simulink model "WTxPSMG3"  (R2023b)
settings: Solver=FixedStepAuto  StartTime=0.0  StopTime=0.2  FixedStep=0.000001  RelTol=1e-3
undefined symbols (not defined in the file): c1, c2, c3, c5, c6, J, Ke, lambda_opt, Ld, Lq, omega_r, p, R, ro, Rs
libraries: slpidlib x1, simulink x1
settings Model: Creator=tudorn  LastModifiedBy=tudorn

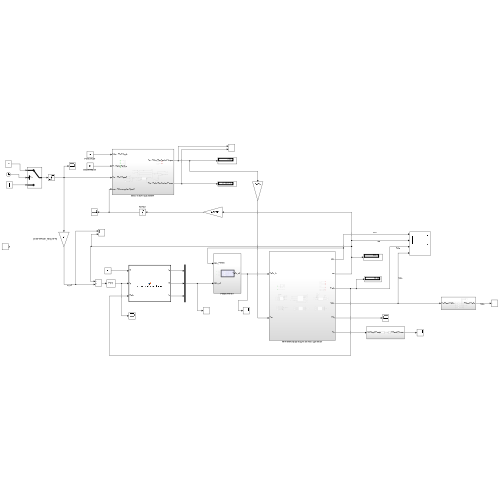
[thumbnail: Simulink's stored preview of the top-level diagram]
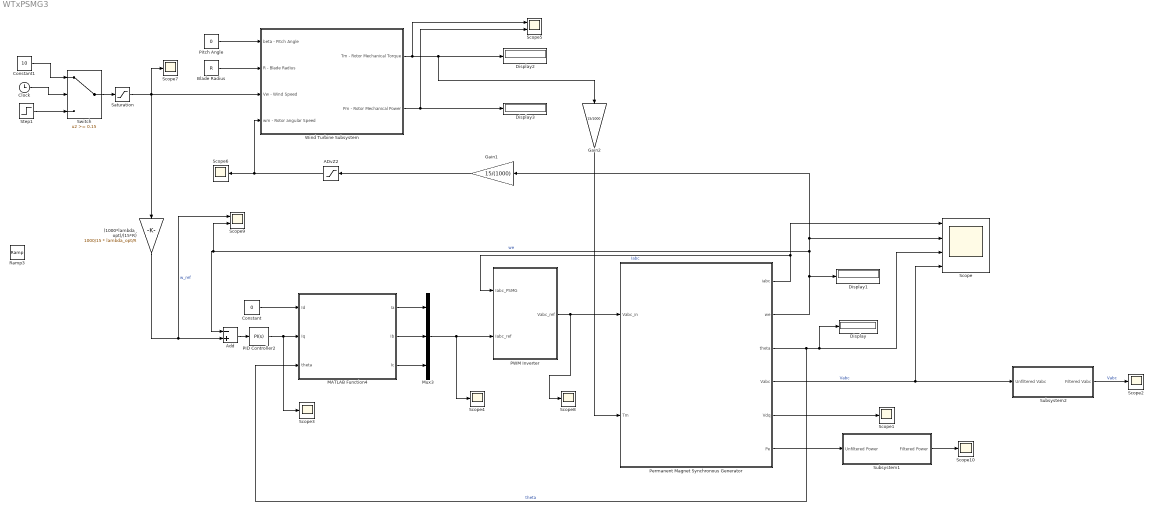
== system WTxPSMG3 ==
  (1000*lambda_opt)/(15*R) : Gain  Gain=1000/15 * lambda_opt/R
  ADvZ2 : Saturate  UpperLimit=omega_r  LowerLimit=1e-6
  Add : Sum  Inputs=-+
  Blade Radius : Constant  Value=R
  Clock : Clock
  Constant : Constant  Value=0
  Constant1 : Constant  Value=10
  Display{,1..3} (4 alike) : Display
  Gain1 : Gain  Gain=15/(1000)
  Gain2 : Gain  Gain=15/1000
  MATLAB Function4 : MATLAB Function  TreatAsAtomicUnit=on
  Mux3 : Mux  Inputs=3
  PID Controller2 : slpidlib/PID Controller  Controller=PI  Form=Parallel  TimeDomain=Continuous-time  UseExternalTs=off  SampleTime=-1  IntegratorMethod=Forward Euler  FilterMethod=Forward Euler  ControllerParametersSource=internal  P=40  I=3  UseKiTs=off  D=0  N=100  UseFilter=on  TunerSelectOption=Transfer Function Based (PID Tuner App)  InitialConditionSource=internal  InitialConditionForIntegrator=0  InitialConditionForFilter=0  DifferentiatorICPrevScaledInput=0  ExternalReset=none  TrackingMode=off  Kt=1  LimitOutput=off  SatLimitsSource=internal  UpperSaturationLimit=inf  LowerSaturationLimit=-inf  LinearizeAsGain=on  AntiWindupMode=none  Kb=1  LimitIntegrator=off  UpperIntegratorSaturationLimit=inf  LowerIntegratorSaturationLimit=-inf  POutMin=[]  POutMax=[]  IOutMin=[]  IOutMax=[]  DOutMin=[]  DOutMax=[]  NOutMin=[]  NOutMax=[]  SumOutMin=[]  SumOutMax=[]  SaturationOutMin=[]  SaturationOutMax=[]  PParamMin=[]  PParamMax=[]  IParamMin=[]  IParamMax=[]  DParamMin=[]  DParamMax=[]  NParamMin=[]  NParamMax=[]  KbParamMin=[]  KbParamMax=[]  KtParamMin=[]  KtParamMax=[]  KbOutMin=[]  KbOutMax=[]  KtOutMin=[]  KtOutMax=[]  IntegratorOutMin=[]  IntegratorOutMax=[]  FilterOutMin=[]  FilterOutMax=[]  SumI1OutMin=[]  SumI1OutMax=[]  SumI2OutMin=[]  SumI2OutMax=[]  SumI3OutMin=[]  SumI3OutMax=[]  SumI4OutMin=[]  SumI4OutMax=[]  SumDOutMin=[]  SumDOutMax=[]  DifferentiatorOutMin=[]  DifferentiatorOutMax=[]  FilterDiffOutCoefMin=[]  FilterDiffOutCoefMax=[]  ReciprocalOutMin=[]  ReciprocalOutMax=[]  SumDenOutMin=[]  SumDenOutMax=[]  SumNumOutMin=[]  SumNumOutMax=[]  DivideOutMin=[]  DivideOutMax=[]  UdiffTsProdOutMin=[]  UdiffTsProdOutMax=[]  NTsProdOutMin=[]  NTsProdOutMax=[]  UintegralTsProdOutMin=[]  UintegralTsProdOutMax=[]  UngainTsProdOutMin=[]  UngainTsProdOutMax=[]  ClampingZeroOutDataTypeStr=Inherit: Inherit via back propagation  ClampingZeroOutMin=[]  ClampingZeroOutMax=[]  FilterDenConstantOutDataTypeStr=Inherit: Inherit via back propagation  FilterDenConstantOutMin=[]  FilterDenConstantOutMax=[]  PCopyOutDataTypeStr=Inherit: Inherit via back propagation  PCopyOutMin=[]  PCopyOutMax=[]  NCopyOutDataTypeStr=Inherit: Inherit via back propagation  NCopyOutMin=[]  NCopyOutMax=[]  IntegratorContinuousStateAttributes=''  IntegratorStateMustResolveToSignalObject=off  IntegratorRTWStateStorageClass=Auto  FilterContinuousStateAttributes=''  FilterStateMustResolveToSignalObject=off  FilterRTWStateStorageClass=Auto  ParallelPVariant=InternalParameters  IdealPVariant=Disabled  IVariant=InternalParameters  DVariant=Disabled  IntegratorVariant=Continuous  SatVariant=Disabled  AWVariant=Passthrough  PCopyVariant=Disabled  TRVariant=Disabled  FdbkBlocksVariant=Forward  IdealPFdbkVariant=Disabled  SatFdbkVariant=Disabled  DerivativeFilterVariant=Disabled  NVariant=Disabled  NCopyVariant=Disabled_SignalSpec  FilterICVariant=Disabled  IntegratorICVariant=InternalICs  ExternalResetVariant=Disabled  TRSumVariant=Passthrough  SumFdbkVariant=Disabled  SumVariant=Sum_PI  TsampFilterVariant=InternalTs  TsampNgainVariant=Passthrough  TsampIntegralVariant=Disabled_SignalSpec  ExternalSaturationOutDataTypeStr=Inherit: Same as second input
  PWM Inverter : Subsystem
  Permanent Magnet Synchronous Generator : Subsystem
  Pitch Angle : Constant  Value=0
  Ramp3 : simulink/Sources/Ramp  slope=100  start=0.02  InitialOutput=7
  Saturation : Saturate  UpperLimit=13  LowerLimit=0
  Scope : Scope  NumInputPorts=4
  Scope{1..4,6..8,10} (8 alike) : Scope
  Scope5 : Scope  NumInputPorts=2
  Scope9 : Scope  NumInputPorts=2
  Step1 : Step  Time=0.075  Before=7  After=12  SampleTime=0
  Subsystem1 : Subsystem
  Subsystem2 : Subsystem
  Switch : Switch  Threshold=0.15  SaturateOnIntegerOverflow=off  InputSameDT=off
  Wind Turbine Subsystem : Subsystem
  wires:
  Gain2/1 -> Permanent Magnet Synchronous Generator/2(Tm)
  PWM Inverter/1(Vabc_ref) -> Scope8/1, Permanent Magnet Synchronous Generator/1(Vabc_in)
  Gain1/1 -> ADvZ2/1
  Blade Radius/1 -> Wind Turbine Subsystem/2(R - Blade Radius)
  MATLAB Function4/1(Ia) -> Mux3/1
  MATLAB Function4/2(Ib) -> Mux3/2
  Constant/1 -> MATLAB Function4/1(Id)
  Pitch Angle/1 -> Wind Turbine Subsystem/1(beta - Pitch Angle)
  Mux3/1 -> Scope4/1, PWM Inverter/2(Iabc_ref)
  Saturation/1 -> Wind Turbine Subsystem/3(Vw - Wind Speed), Scope7/1, (1000*lambda_opt)/(15*R)/1
  Wind Turbine Subsystem/2(Pm - Rotor Mechanical Power) -> Display3/1, Scope5/2
  Wind Turbine Subsystem/1(Tm - Rotor Mechanical Torque) -> Gain2/1, Display2/1, Scope5/1
  Permanent Magnet Synchronous Generator/1(iabc) -> Scope/1, PWM Inverter/1(Iabc_PSMG)  "Iabc"
  MATLAB Function4/3(Ic) -> Mux3/3
  Permanent Magnet Synchronous Generator/3(theta) -> MATLAB Function4/3(theta), Display/1, Scope/3  "theta"
  Permanent Magnet Synchronous Generator/2(we) -> Scope9/2, Add/1, Scope/2, Gain1/1, Display1/1  "we"
  (1000*lambda_opt)/(15*R)/1 -> Add/2, Scope9/1  "w_ref"
  Permanent Magnet Synchronous Generator/5(Vdq) -> Scope1/1
  ADvZ2/1 -> Scope6/1, Wind Turbine Subsystem/4(wm - Rotor angular Speed)
  Permanent Magnet Synchronous Generator/4(Vabc) -> Subsystem2/1(Unfiltered Vabc), Scope/4  "Vabc"
  Add/1 -> PID Controller2/1
  PID Controller2/1 -> Scope3/1, MATLAB Function4/2(Iq)
  Permanent Magnet Synchronous Generator/6(Pe) -> Subsystem1/1(Unfiltered Power)
  Subsystem2/1(Filtered Vabc) -> Scope2/1  "Vabc"
  Subsystem1/1(Filtered Power) -> Scope10/1
  Switch/1 -> Saturation/1
  Constant1/1 -> Switch/1
  Step1/1 -> Switch/3
  Clock/1 -> Switch/2

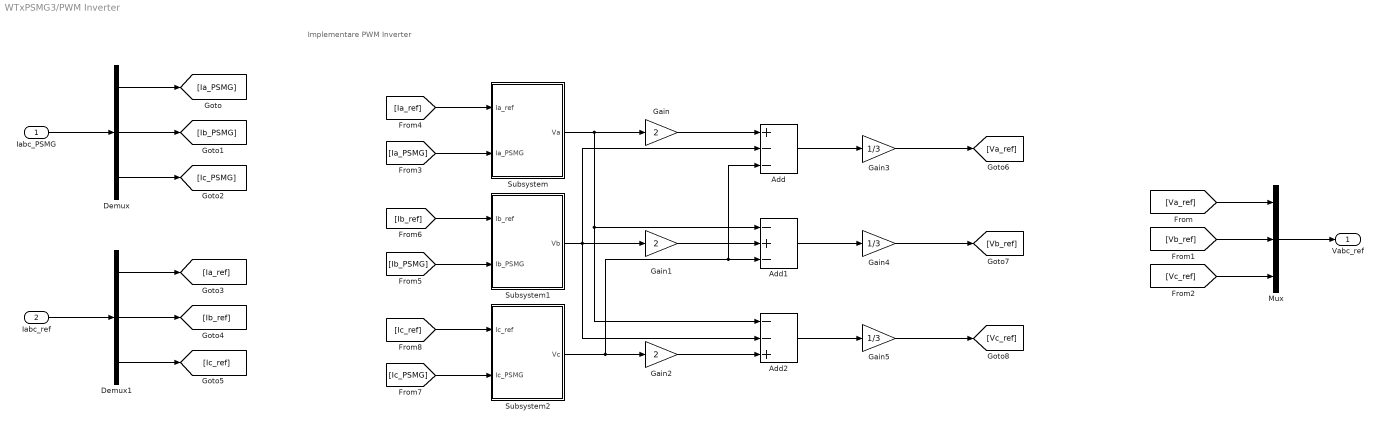
== system WTxPSMG3/PWM Inverter ==
  note: Implementare PWM Inverter
  Iabc_PSMG : Inport
  Iabc_ref : Inport  Port=2
  Add : Sum  Inputs=+--
  Add1 : Sum  Inputs=-+-
  Add2 : Sum  Inputs=--+
  Demux : Demux  Outputs=3
  Demux1 : Demux  Outputs=3
  Gain : Gain  Gain=2
  Gain1 : Gain  Gain=2
  Gain2 : Gain  Gain=2
  Gain3 : Gain  Gain=1/3
  Gain4 : Gain  Gain=1/3
  Gain5 : Gain  Gain=1/3
  Mux : Mux  Inputs=3
  Subsystem : Subsystem
  Subsystem1 : Subsystem
  Subsystem2 : Subsystem
  Vabc_ref : Outport
  wires:
  Iabc_PSMG/1 -> Demux/1
  Mux/1 -> Vabc_ref/1
  Demux/1 -> [Ia_PSMG]
  Demux/2 -> [Ib_PSMG]
  Demux/3 -> [Ic_PSMG]
  Demux1/3 -> [Ic_ref]
  Demux1/2 -> [Ib_ref]
  Demux1/1 -> [Ia_ref]
  Iabc_ref/1 -> Demux1/1
  [Va_ref] -> Mux/1
  [Vb_ref] -> Mux/2
  [Vc_ref] -> Mux/3
  [Ia_ref] -> Subsystem/1(Ia_ref)
  [Ia_PSMG] -> Subsystem/2(Ia_PSMG)
  [Ib_ref] -> Subsystem1/1(Ib_ref)
  [Ib_PSMG] -> Subsystem1/2(Ib_PSMG)
  [Ic_ref] -> Subsystem2/1(Ic_ref)
  [Ic_PSMG] -> Subsystem2/2(Ic_PSMG)
  Subsystem/1(Va) -> Add2/1, Add1/1, Gain/1
  Subsystem2/1(Vc) -> Add/3, Add1/3, Gain2/1
  Subsystem1/1(Vb) -> Add2/2, Gain1/1, Add/2
  Gain/1 -> Add/1
  Gain1/1 -> Add1/2
  Gain2/1 -> Add2/3
  Add/1 -> Gain3/1
  Add1/1 -> Gain4/1
  Add2/1 -> Gain5/1
  Gain5/1 -> [Vc_ref]
  Gain4/1 -> [Vb_ref]
  Gain3/1 -> [Va_ref]

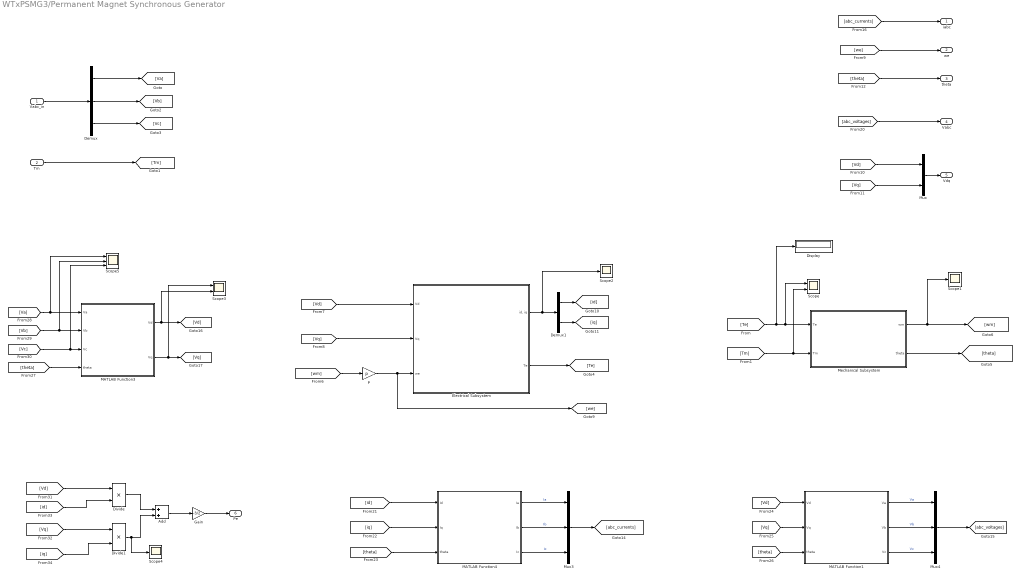
== system WTxPSMG3/Permanent Magnet Synchronous Generator ==
  Vabc_in : Inport
  Tm : Inport  Port=2
  Add : Sum
  Demux : Demux  Outputs=3
  Demux1 : Demux  Outputs=2
  Display : Display
  Divide : Product  Inputs=**
  Divide1 : Product  Inputs=**
  Electrical Subsystem : Subsystem
  Gain : Gain  Gain=-3/2
  MATLAB Function1 : MATLAB Function  TreatAsAtomicUnit=on
  MATLAB Function3 : MATLAB Function  TreatAsAtomicUnit=on
  MATLAB Function4 : MATLAB Function  TreatAsAtomicUnit=on
  Mechanical Subsystem : Subsystem
  Mux : Mux  Inputs=2
  Mux3 : Mux  Inputs=3
  Mux4 : Mux  Inputs=3
  P : Gain  Gain=p
  Scope : Scope  NumInputPorts=2
  Scope1 : Scope
  Scope2 : Scope
  Scope3 : Scope  NumInputPorts=2
  Scope4 : Scope
  Scope5 : Scope  NumInputPorts=3
  iabc : Outport
  we : Outport  Port=2
  theta : Outport  Port=3
  Vabc : Outport  Port=4
  Vdq : Outport  Port=5
  Pe : Outport  Port=6
  wires:
  Vabc_in/1 -> Demux/1
  Tm/1 -> [Tm]
  Demux/1 -> [Va]
  Demux/2 -> [Vb]
  Demux/3 -> [Vc]
  Electrical Subsystem/2(Te) -> [Te]
  [Te] -> Display/1, Scope/1, Mechanical Subsystem/1(Te)
  [Tm] -> Scope/2, Mechanical Subsystem/2(Tm)
  Mechanical Subsystem/1(wm) -> Scope1/1, [wm]
  [wm] -> P/1
  P/1 -> [we], Electrical Subsystem/3(we)
  [Vq] -> Electrical Subsystem/2(Vq)
  [Vd] -> Electrical Subsystem/1(Vd)
  [we] -> we/1
  Mux/1 -> Vdq/1
  [Vd] -> Mux/1
  [Vq] -> Mux/2
  [theta] -> theta/1
  Electrical Subsystem/1("id, iq") -> Scope2/1, Demux1/1
  Demux1/1 -> [id]
  Demux1/2 -> [iq]
  [abc_currents] -> iabc/1
  [abc_voltages] -> Vabc/1
  [iq] -> MATLAB Function4/2(Iq)
  [theta] -> MATLAB Function4/3(theta)
  [id] -> MATLAB Function4/1(Id)
  Mux3/1 -> [abc_currents]
  MATLAB Function4/2(Ib) -> Mux3/2  "Ib"
  MATLAB Function4/1(Ia) -> Mux3/1  "Ia"
  MATLAB Function4/3(Ic) -> Mux3/3  "Ic"
  [Vd] -> MATLAB Function1/1(Vd)
  [Vq] -> MATLAB Function1/2(Vq)
  [theta] -> MATLAB Function1/3(theta)
  Mux4/1 -> [abc_voltages]
  MATLAB Function1/1(Va) -> Mux4/1  "Va"
  MATLAB Function1/2(Vb) -> Mux4/2  "Vb"
  MATLAB Function1/3(Vc) -> Mux4/3  "Vc"
  [Va] -> Scope5/1, MATLAB Function3/1(Va)
  [Vc] -> Scope5/3, MATLAB Function3/3(Vc)
  [theta] -> MATLAB Function3/4(theta)
  [Vb] -> Scope5/2, MATLAB Function3/2(Vb)
  MATLAB Function3/2(Vq) -> Scope3/1, [Vq]
  MATLAB Function3/1(Vd) -> Scope3/2, [Vd]
  [Vq] -> Divide1/1
  [iq] -> Divide1/2
  [id] -> Divide/2
  [Vd] -> Divide/1
  Divide/1 -> Add/1
  Divide1/1 -> Scope4/1, Add/2
  Add/1 -> Gain/1
  Gain/1 -> Pe/1
  Mechanical Subsystem/2(theta) -> [theta]

== system WTxPSMG3/Subsystem1 ==
  Unfiltered Power : Inport
  Saturation : Saturate  UpperLimit=4500  LowerLimit=-45
  Transfer Fcn : TransferFcn  Denominator=[1e-2 1]
  Filtered Power : Outport
  wires:
  Transfer Fcn/1 -> Saturation/1
  Unfiltered Power/1 -> Transfer Fcn/1
  Saturation/1 -> Filtered Power/1

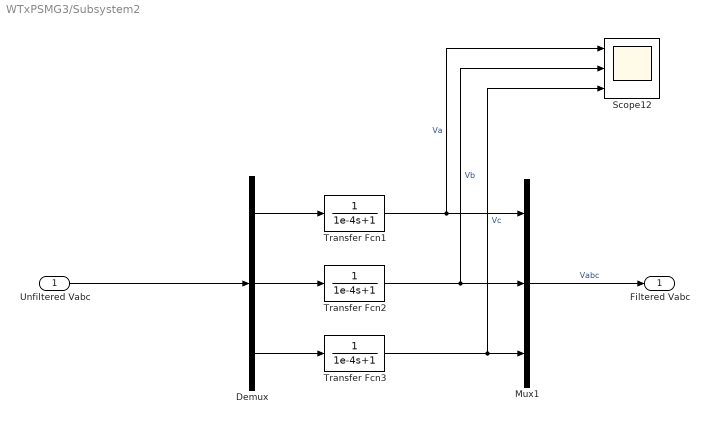
== system WTxPSMG3/Subsystem2 ==
  Unfiltered Vabc : Inport
  Demux : Demux  Outputs=3
  Mux1 : Mux  Inputs=3
  Scope12 : Scope  NumInputPorts=3
  Transfer Fcn1 : TransferFcn  Numerator=1  Denominator=[1e-4 1]
  Transfer Fcn2 : TransferFcn  Numerator=1  Denominator=[1e-4 1]
  Transfer Fcn3 : TransferFcn  Numerator=1  Denominator=[1e-4 1]
  Filtered Vabc : Outport
  wires:
  Demux/3 -> Transfer Fcn3/1
  Transfer Fcn3/1 -> Scope12/3, Mux1/3  "Vc"
  Demux/2 -> Transfer Fcn2/1
  Demux/1 -> Transfer Fcn1/1
  Transfer Fcn1/1 -> Scope12/1, Mux1/1  "Va"
  Transfer Fcn2/1 -> Scope12/2, Mux1/2  "Vb"
  Unfiltered Vabc/1 -> Demux/1
  Mux1/1 -> Filtered Vabc/1  "Vabc"

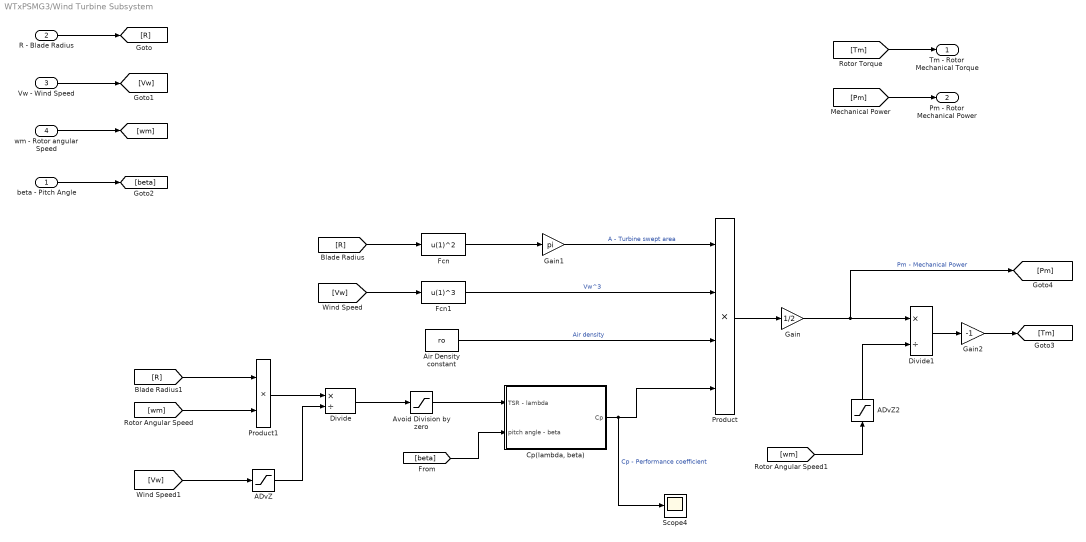
== system WTxPSMG3/Wind Turbine Subsystem ==
  beta - Pitch Angle : Inport
  R - Blade Radius : Inport  Port=2
  Vw - Wind Speed : Inport  Port=3
  wm - Rotor angular Speed : Inport  Port=4
  ADvZ : Saturate  UpperLimit=1e6  LowerLimit=1e-6
  ADvZ2 : Saturate  UpperLimit=omega_r  LowerLimit=1e-6
  Air Density constant : Constant  Value=ro
  Avoid Division by zero : Saturate  UpperLimit=Inf  LowerLimit=1e-6
  "Cp(lambda, beta)" : Subsystem
  Divide : Product  Inputs=*/
  Divide1 : Product  Inputs=*/
  Fcn : Fcn  Expr=u(1)^2
  Fcn1 : Fcn  Expr=u(1)^3
  Gain : Gain  Gain=1/2
  Gain1 : Gain  Gain=pi
  Gain2 : Gain  Gain=-1
  Product : Product  Inputs=4
  Product1 : Product
  Scope4 : Scope
  Tm - Rotor Mechanical Torque : Outport
  Pm - Rotor Mechanical Power : Outport  Port=2
  wires:
  Product/1 -> Gain/1
  Gain1/1 -> Product/1  "A - Turbine swept area"
  Fcn1/1 -> Product/2  "Vw^3"
  Air Density constant/1 -> Product/3  "Air density"
  "Cp(lambda, beta)"/1(Cp) -> Scope4/1, Product/4  "Cp - Performance coefficient"
  Fcn/1 -> Gain1/1
  R - Blade Radius/1 -> [R]
  Vw - Wind Speed/1 -> [Vw]
  [R] -> Fcn/1
  [Vw] -> Fcn1/1
  wm - Rotor angular Speed/1 -> [wm]
  [R] -> Product1/1
  [wm] -> Product1/2
  Product1/1 -> Divide/1
  [Vw] -> ADvZ/1
  Divide/1 -> Avoid Division by zero/1
  ADvZ/1 -> Divide/2
  beta - Pitch Angle/1 -> [beta]
  [beta] -> "Cp(lambda, beta)"/2(pitch angle - beta)
  [Tm] -> Tm - Rotor Mechanical Torque/1
  Gain/1 -> Divide1/1, [Pm]  "Pm - Mechanical Power"
  Divide1/1 -> Gain2/1
  [wm] -> ADvZ2/1
  [Pm] -> Pm - Rotor Mechanical Power/1
  ADvZ2/1 -> Divide1/2
  Avoid Division by zero/1 -> "Cp(lambda, beta)"/1(TSR - lambda)
  Gain2/1 -> [Tm]

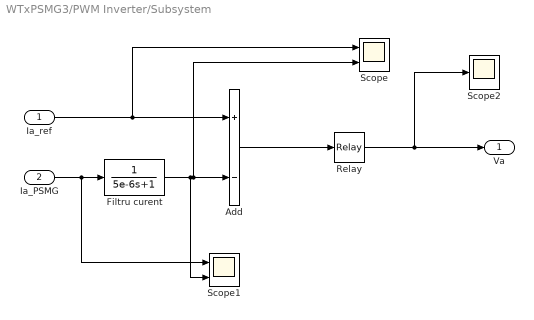
== system WTxPSMG3/PWM Inverter/Subsystem ==
  Ia_ref : Inport
  Ia_PSMG : Inport  Port=2
  Add : Sum  Inputs=+-
  Filtru curent : TransferFcn  Denominator=[5e-6 1]
  Relay : Relay  OnSwitchValue=0.05  OffSwitchValue=-0.05  OnOutputValue=155  OffOutputValue=-155
  Scope : Scope  NumInputPorts=2
  Scope1 : Scope  NumInputPorts=2
  Scope2 : Scope
  Va : Outport
  wires:
  Ia_ref/1 -> Scope/1, Add/1
  Ia_PSMG/1 -> Filtru curent/1, Scope1/1
  Filtru curent/1 -> Scope1/2, Scope/2, Add/2
  Add/1 -> Relay/1
  Relay/1 -> Scope2/1, Va/1

== system WTxPSMG3/PWM Inverter/Subsystem1 ==
  Ib_ref : Inport
  Ib_PSMG : Inport  Port=2
  Add : Sum  Inputs=+-
  Filtru curent : TransferFcn  Denominator=[5e-6 1]
  Relay : Relay  OnSwitchValue=0.05  OffSwitchValue=-0.05  OnOutputValue=155  OffOutputValue=-155
  Vb : Outport
  wires:
  Relay/1 -> Vb/1
  Add/1 -> Relay/1
  Filtru curent/1 -> Add/2
  Ib_PSMG/1 -> Filtru curent/1
  Ib_ref/1 -> Add/1

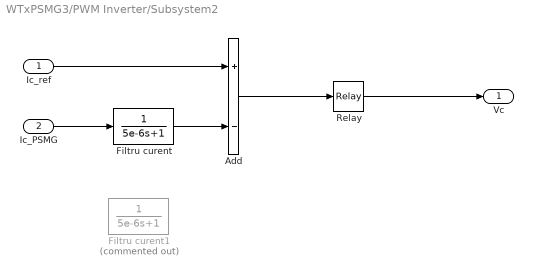
== system WTxPSMG3/PWM Inverter/Subsystem2 ==
  Ic_ref : Inport
  Ic_PSMG : Inport  Port=2
  Add : Sum  Inputs=+-
  Filtru curent : TransferFcn  Denominator=[5e-6 1]
  Filtru curent1 : TransferFcn  Commented=on  Denominator=[5e-6 1]
  Relay : Relay  OnSwitchValue=0.05  OffSwitchValue=-0.05  OnOutputValue=155  OffOutputValue=-155
  Vc : Outport
  wires:
  Ic_ref/1 -> Add/1
  Ic_PSMG/1 -> Filtru curent/1
  Add/1 -> Relay/1
  Relay/1 -> Vc/1
  Filtru curent/1 -> Add/2

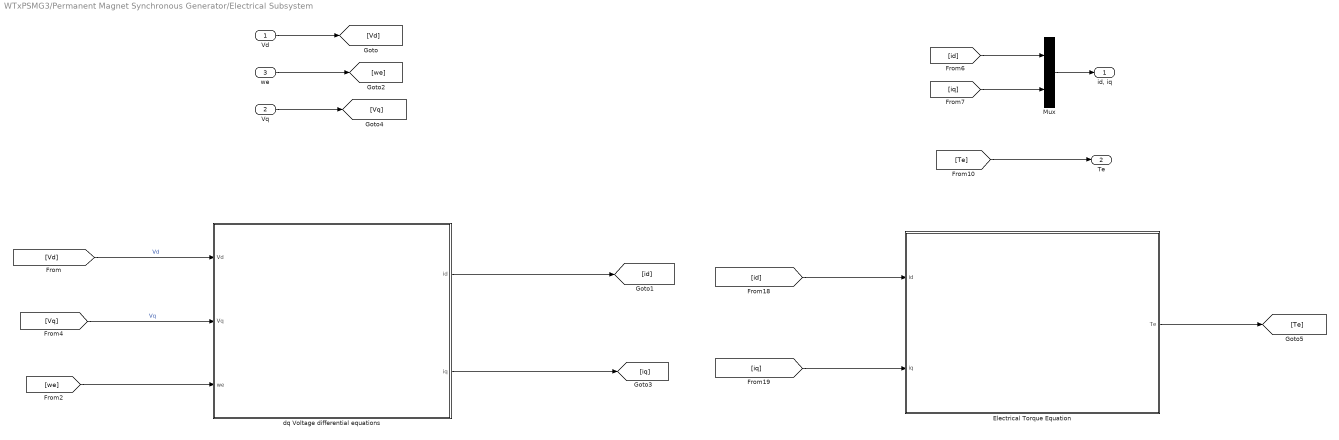
== system WTxPSMG3/Permanent Magnet Synchronous Generator/Electrical Subsystem ==
  Vd : Inport
  Vq : Inport  Port=2
  we : Inport  Port=3
  Electrical Torque Equation : Subsystem
  Mux : Mux  Inputs=2
  dq Voltage differential equations : Subsystem
  "id, iq" : Outport
  Te : Outport  Port=2
  wires:
  Vd/1 -> [Vd]
  we/1 -> [we]
  Vq/1 -> [Vq]
  Mux/1 -> "id, iq"/1
  [id] -> Mux/1
  [iq] -> Mux/2
  [Te] -> Te/1
  [Vd] -> dq Voltage differential equations/1(Vd)  "Vd"
  [Vq] -> dq Voltage differential equations/2(Vq)  "Vq"
  dq Voltage differential equations/1(id) -> [id]
  dq Voltage differential equations/2(iq) -> [iq]
  [id] -> Electrical Torque Equation/1(id)
  [iq] -> Electrical Torque Equation/2(iq)
  Electrical Torque Equation/1(Te) -> [Te]
  [we] -> dq Voltage differential equations/3(we)

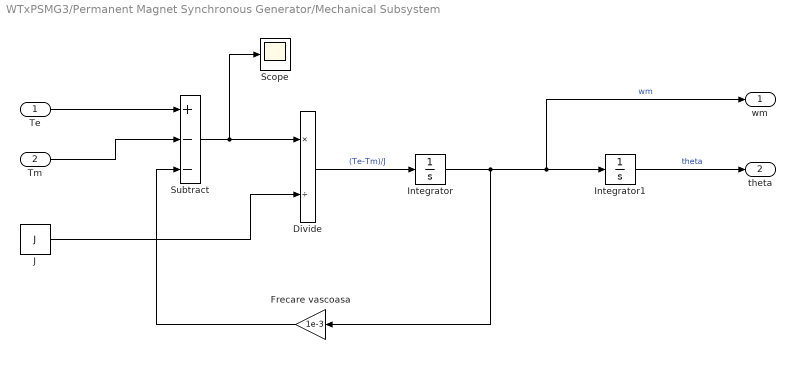
== system WTxPSMG3/Permanent Magnet Synchronous Generator/Mechanical Subsystem ==
  Te : Inport
  Tm : Inport  Port=2
  Divide : Product  Inputs=*/
  Frecare vascoasa : Gain  Gain=1e-3
  Integrator : Integrator
  Integrator1 : Integrator
  J : Constant  Value=J
  Scope : Scope
  Subtract : Sum  Inputs=+--
  wm : Outport
  theta : Outport  Port=2
  wires:
  Te/1 -> Subtract/1
  Subtract/1 -> Scope/1, Divide/1
  J/1 -> Divide/2
  Divide/1 -> Integrator/1  "(Te-Tm)/J"
  Integrator/1 -> Frecare vascoasa/1, Integrator1/1, wm/1  "wm"
  Integrator1/1 -> theta/1  "theta"
  Frecare vascoasa/1 -> Subtract/3
  Tm/1 -> Subtract/2

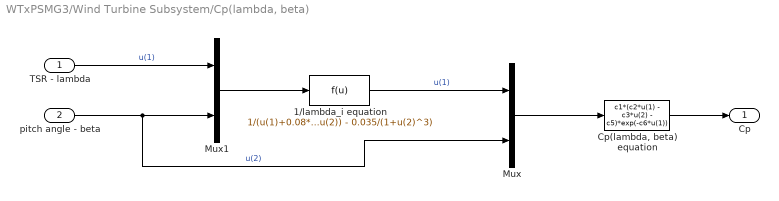
== system WTxPSMG3/Wind Turbine Subsystem/Cp(lambda, beta) ==
  TSR - lambda : Inport
  pitch angle - beta : Inport  Port=2
  1/lambda_i equation : Fcn  Expr=1/(u(1)+0.08*u(2)) - 0.035/(1+u(2)^3)
  "Cp(lambda, beta) equation" : Fcn  Expr=c1*(c2*u(1) - c3*u(2) - c5)*exp(-c6*u(1))
  Mux : Mux  Inputs=2
  Mux1 : Mux  Inputs=2
  Cp : Outport
  wires:
  "Cp(lambda, beta) equation"/1 -> Cp/1
  Mux/1 -> "Cp(lambda, beta) equation"/1
  1/lambda_i equation/1 -> Mux/1  "u(1)"
  pitch angle - beta/1 -> Mux/2, Mux1/2  "u(2)"
  Mux1/1 -> 1/lambda_i equation/1
  TSR - lambda/1 -> Mux1/1  "u(1)"

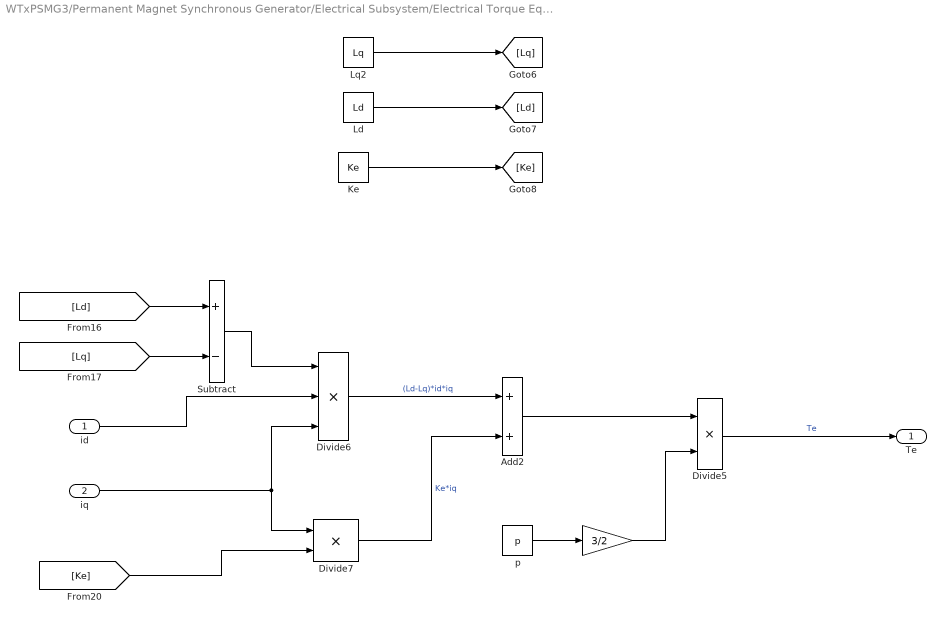
== system WTxPSMG3/Permanent Magnet Synchronous Generator/Electrical Subsystem/Electrical Torque Equation ==
  id : Inport
  iq : Inport  Port=2
  " " : Gain  Gain=3/2
  Add2 : Sum
  Divide5 : Product  Inputs=**
  Divide6 : Product  Inputs=***
  Divide7 : Product  Inputs=**
  Ke : Constant  Value=Ke
  Ld : Constant  Value=Ld
  Lq2 : Constant  Value=Lq
  Subtract : Sum  Inputs=+-
  p : Constant  Value=p
  Te : Outport
  wires:
  id/1 -> Divide6/2
  [Ke] -> Divide7/2
  Divide5/1 -> Te/1  "Te"
  " "/1 -> Divide5/2
  iq/1 -> Divide7/1, Divide6/3
  [Ld] -> Subtract/1
  Subtract/1 -> Divide6/1
  p/1 -> " "/1
  Add2/1 -> Divide5/1
  Divide6/1 -> Add2/1  "(Ld-Lq)*id*iq"
  [Lq] -> Subtract/2
  Divide7/1 -> Add2/2  "Ke*iq"
  Ld/1 -> [Ld]
  Lq2/1 -> [Lq]
  Ke/1 -> [Ke]

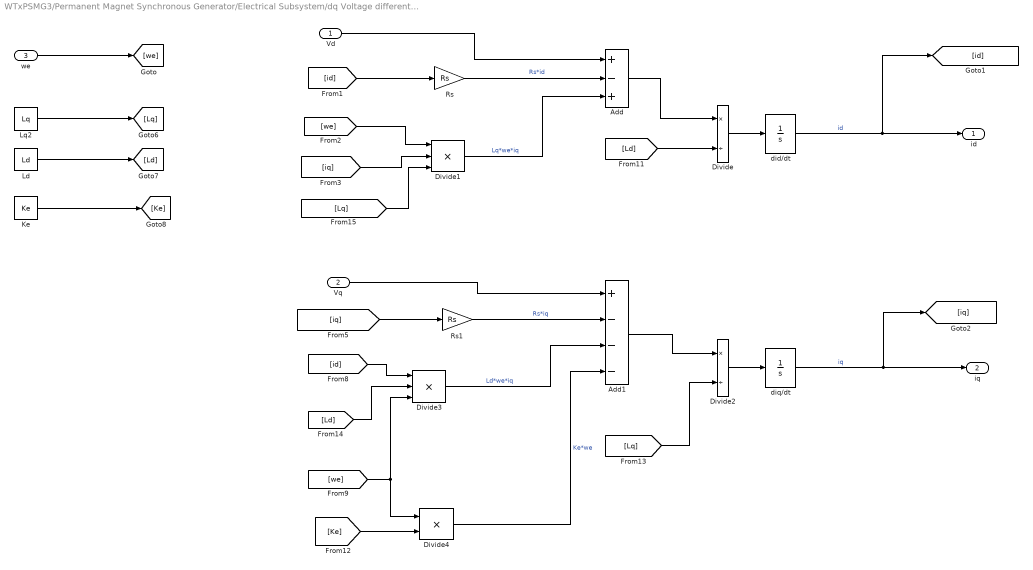
== system WTxPSMG3/Permanent Magnet Synchronous Generator/Electrical Subsystem/dq Voltage differential equations ==
  Vd : Inport
  Vq : Inport  Port=2
  we : Inport  Port=3
  Add : Sum  Inputs=+-+
  Add1 : Sum  Inputs=+---
  Divide : Product  Inputs=*/
  Divide1 : Product  Inputs=***
  Divide2 : Product  Inputs=*/
  Divide3 : Product  Inputs=***
  Divide4 : Product  Inputs=**
  Ke : Constant  Value=Ke
  Ld : Constant  Value=Ld
  Lq2 : Constant  Value=Lq
  Rs : Gain  Gain=Rs
  Rs1 : Gain  Gain=Rs
  did/dt : Integrator
  diq/dt : Integrator
  id : Outport
  iq : Outport  Port=2
  wires:
  diq/dt/1 -> [iq], iq/1  "iq"
  Add/1 -> Divide/1
  did/dt/1 -> [id], id/1  "id"
  Rs1/1 -> Add1/2  "Rs*iq"
  [Lq] -> Divide2/2
  Vq/1 -> Add1/1
  [iq] -> Divide1/2
  [id] -> Divide3/1
  Divide1/1 -> Add/3  "Lq*we*iq"
  Add1/1 -> Divide2/1
  [iq] -> Rs1/1
  [Ld] -> Divide3/2
  Divide2/1 -> diq/dt/1
  [Lq] -> Divide1/3
  Rs/1 -> Add/2  "Rs*id"
  [we] -> Divide1/1
  Divide/1 -> did/dt/1
  [Ke] -> Divide4/2
  [we] -> Divide3/3, Divide4/1
  Divide4/1 -> Add1/4  "Ke*we"
  Divide3/1 -> Add1/3  "Ld*we*iq"
  [id] -> Rs/1
  Vd/1 -> Add/1
  [Ld] -> Divide/2
  Ld/1 -> [Ld]
  Lq2/1 -> [Lq]
  Ke/1 -> [Ke]
  we/1 -> [we]

== matlab function WTxPSMG3/Permanent Magnet Synchronous Generator/MATLAB Function1 ==
  data: Vd input; Va output; Vq input; theta input; Vb output; Vc output
function [Va, Vb, Vc] = Inverse_ClarkePark_Voltage(Vd, Vq, theta)

    if isempty(theta)
        theta = 0;
    end

    Valpha = Vd .* cos(theta) - Vq .* sin(theta);
    Vbeta = Vd .* sin(theta) + Vq .* cos(theta);

    Va = Valpha;
    Vb = Valpha * (-1)/2 + Vbeta * sqrt(3)/2;
    Vc = Valpha * (-1)/2 - Vbeta * sqrt(3)/2;



end

== matlab function WTxPSMG3/Permanent Magnet Synchronous Generator/MATLAB Function3 ==
  data: Va input; Vd output; Vb input; Vc input; theta input; Vq output
function [Vd, Vq] = ClarkePark(Va, Vb, Vc, theta)

    if isempty(theta)
        theta = 0;
    end
    
    Valpha = 2/3 * (Va - 0.5 * Vb - 0.5 * Vc);
    Vbeta = 2/3 * (sqrt(3)/2 * Vb - sqrt(3)/2 * Vc);

    Vd = Valpha .* cos(theta) + Vbeta .* sin(theta);
    Vq = -Valpha .* sin(theta) + Vbeta .* cos(theta);

end

== matlab function WTxPSMG3/MATLAB Function4 ==
  data: Id input; Ia output; Iq input; theta input; Ib output; Ic output
function [Ia, Ib, Ic] = Inverse_ClarkePark_Current(Id, Iq, theta)

    if isempty(theta)
        theta = 0;
    end

    Ialpha = Id .* cos(theta) - Iq .* sin(theta);
    Ibeta = Id .* sin(theta) + Iq .* cos(theta);

    Ia = Ialpha;
    Ib = Ialpha * (-1)/2 + Ibeta * sqrt(3)/2;
    Ic = Ialpha * (-1)/2 - Ibeta * sqrt(3)/2;


end

== matlab function WTxPSMG3/Permanent Magnet Synchronous Generator/MATLAB Function4 ==
  data: Id input; Ia output; Iq input; theta input; Ib output; Ic output
function [Ia, Ib, Ic] = Inverse_ClarkePark_Current(Id, Iq, theta)

    if isempty(theta)
        theta = 0;
    end

    Ialpha = Id .* cos(theta) - Iq .* sin(theta);
    Ibeta = Id .* sin(theta) + Iq .* cos(theta);

    Ia = Ialpha;
    Ib = Ialpha * (-1)/2 + Ibeta * sqrt(3)/2;
    Ic = Ialpha * (-1)/2 - Ibeta * sqrt(3)/2;


end
